simulink model "week1_project1_simu"  (R2020a)
settings: Solver=VariableStepAuto  StartTime=0.0  StopTime=10  MaxStep=0.01  RelTol=1e-3
model workspace (MAT data in the model file):
  M1 = Simulink.Parameter
  M1.Value = 100
  M1.Description = 'mass'
  M1.DataType = 'auto'
  M1.Dimensions = [1 1]
  M2 = Simulink.Parameter
  M2.Value = 95
  M2.Description = 'mass
    | '
  M2.DataType = 'auto'
  M2.Dimensions = [1 1]
  b = Simulink.Parameter
  b.Value = 50
  b.Description = 'damping coefficient'
  b.DataType = 'auto'
  b.Dimensions = [1 1]
  k1 = Simulink.Parameter
  k1.Value = 50
  k1.Description = 'spring constant'
  k1.DataType = 'auto'
  k1.Dimensions = [1 1]
  k12 = Simulink.Parameter
  k12.Value = 9500
  k12.DataType = 'auto'
  k12.Dimensions = [1 1]
settings Model: OrderedModelArguments=off  Creator=DELL  LastModifiedBy=DELL

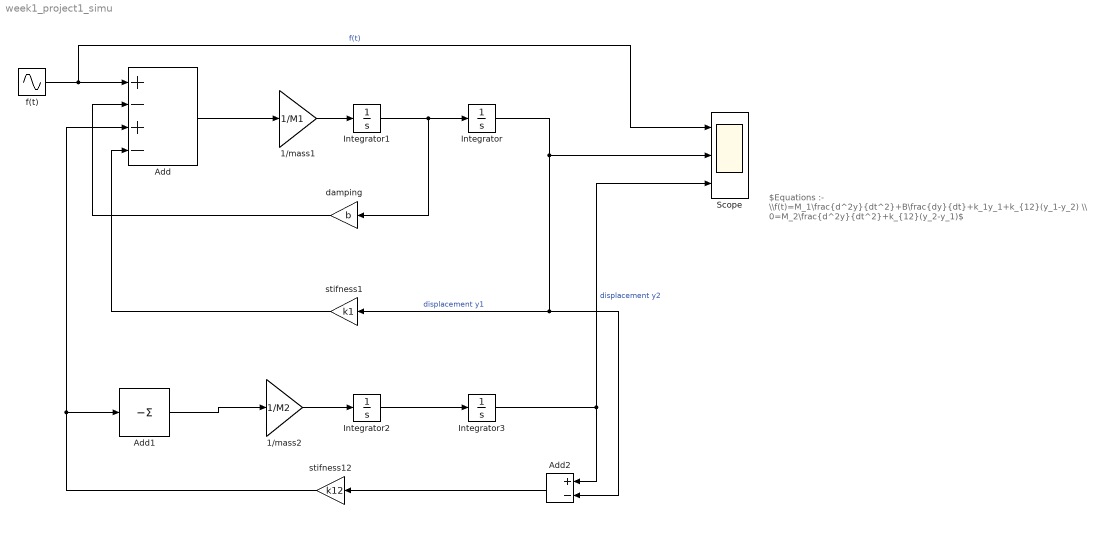
== system week1_project1_simu ==
  note: $Equations :- \\f(t)=M_1\frac{d^2y}{dt^2}+B\frac{dy}{dt}+k_1y_1+k_{12}(y_1-y_2) \\ 0=M_2\frac{d^2y}{dt^2}+k_{12}(y_2-y_1)$
  1/mass1 : Gain  Gain=1/M1
  1/mass2 : Gain  Gain=1/M2
  Add : Sum  Inputs=+-+-
  Add1 : Sum  Inputs=-
  Add2 : Sum  Inputs=+-
  Integrator{,1..3} (4 alike) : Integrator
  Scope : Scope  NumInputPorts=3
  damping : Gain  Gain=b
  f(t) : Sin  Amplitude=2  Frequency=10  SampleTime=0
  stifness1 : Gain  Gain=k1
  stifness12 : Gain  Gain=k12
  wires:
  f(t)/1 -> Scope/1, Add/1  "f(t)"
  Add/1 -> 1/mass1/1
  Integrator1/1 -> damping/1, Integrator/1
  1/mass1/1 -> Integrator1/1
  stifness1/1 -> Add/4
  damping/1 -> Add/2
  Integrator/1 -> Scope/2, Add2/2, stifness1/1  "displacement y1"
  1/mass2/1 -> Integrator2/1
  Add1/1 -> 1/mass2/1
  Integrator2/1 -> Integrator3/1
  Integrator3/1 -> Add2/1, Scope/3  "displacement y2"
  stifness12/1 -> Add1/1, Add/3
  Add2/1 -> stifness12/1
